simulink model "PMSM_motor"  (R2025b)
settings: Solver=VariableStepAuto  StartTime=0.0  StopTime=10  RelTol=1e-3
values from neighbouring files (symbols this model uses):
  p = 3    [task_run.m]    (also in task_run1.m; task_run2.m)
undefined symbols (not defined in the file or in its folder): Ld, Lq, omega_m_const, psi_f, Rs, theta_offset
libraries: fl_lib x10, nesl_utility x6, ee_lib x4
settings Model: Creator=Администратор  LastModifiedBy=Администратор

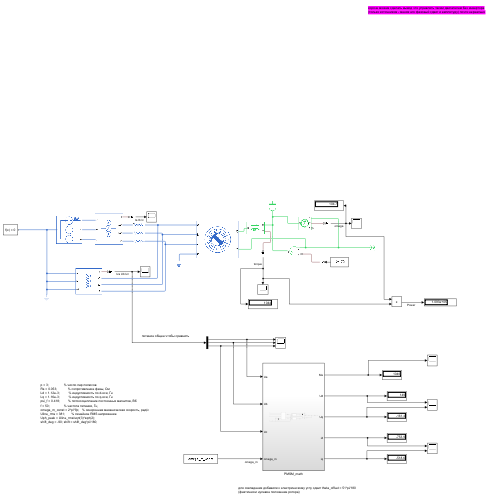
[thumbnail: Simulink's stored preview of the top-level diagram]
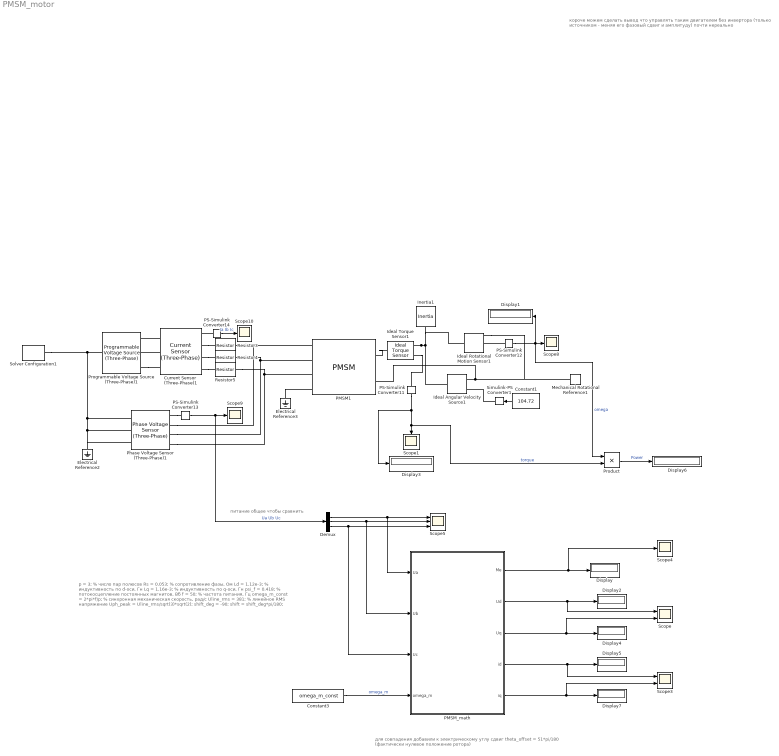
== system PMSM_motor ==
  note: для совпадения добавили к электрическому углу сдвиг theta_offset = 51*pi/180 (фактически нулевое положение ротора)
  note: питание общее чтобы сравнить
  note: p = 3;                 % число пар полюсов
      | Rs = 0.053;            % сопротивление фазы, Ом
      | Ld = 1.12e-3;          % индуктивность по d-оси, Гн
      | Lq = 1.16e-3;          % индуктивность по q-оси, Гн
      | psi_f = 0.418;         % потокосцепление постоянных магнитов, Вб
      | f = 50;                % частота питания, Гц
      | omega_m_const = 2*pi*f/p;   % синхронная механическая скорость, рад/с
      | Uline_rms = 381;       % линейное RMS напряжение
      | Uph_peak = Uline_rms/sqrt(3)*sqrt(2);
      | shift_deg = -90; shift = shift_deg*pi/180;
  note: короче можем сделать вывод что управлять таким двигателем без инвертора
      | (только источником - меняя его фазовый сдвиг и амплитуду) почти нереально
  Constant1 : Constant  Value=104.72
  Constant3 : Constant  Value=omega_m_const
  Current Sensor (Three-Phase)1 : ee_lib/Sensors & Transducers/Current Sensor (Three-Phase)
      settings: InternalSimscapePortConfiguration="{\"Bottom\":[],\"Left\":[{\"id\":\"a1\",\"label\":\"a1\",\"type\":\"foundation.electrical.electrical\"},{\"id\":\"b1\",\"label\":\"b1\",\"type\":\"foundation.electrical.electrical\"},{\"id\":\"c1\",\"label\":\"c1\",\"type\":\"foundation.electrical.electrical\"}],\"Right\":[{\"id\":\"I_output\",\"label\":\"I\",\"type\":\"output\"},{\"id\":\"a2\",\"label\":\"a2\",\"type\":\"foundation.electrical.electrical\"},{\"id\":\"b2\",\"label\":\"b2\",\"type\":\"foundation.electrical.electrical\"},{\"id\":\"c2\",\"label\":\"c2\",\"type\":\"foundation.electrical.electrical\"}],\"Top\":[]}"
  Demux : Demux  Outputs=3
  Display{,1..7} (8 alike) : Display
  Electrical Reference2 : fl_lib/Electrical/Electrical Elements/Electrical Reference
  Electrical Reference3 : fl_lib/Electrical/Electrical Elements/Electrical Reference
  Ideal Angular Velocity Source1 : fl_lib/Mechanical/Mechanical Sources/Ideal Angular Velocity Source
  Ideal Rotational Motion Sensor1 : fl_lib/Mechanical/Mechanical Sensors/Ideal Rotational Motion Sensor  reference=foundation.enum.MeasurementReference.difference  acceleration_port=false  velocity_port=true  position_port=true  wrap_angle=false  offset=0 rad
  Ideal Torque Sensor1 : fl_lib/Mechanical/Mechanical Sensors/Ideal Torque Sensor
  Inertia1 : fl_lib/Mechanical/Rotational Elements/Inertia  inertia=0.05 kg*m^2  num_ports=foundation.enum.numPorts2.one  w_specify=off  w_priority=High  w=0 rad/s  w_nominal_specify=off  w_nominal_value=1  w_nominal_unit=rad/s  t_specify=off  t_priority=None  t=0 N*m  t_nominal_specify=off  t_nominal_value=1  t_nominal_unit=N*m
  Mechanical Rotational Reference1 : fl_lib/Mechanical/Rotational Elements/Mechanical Rotational Reference
  PMSM1 : ee_lib/Electromechanical/Permanent Magnet/PMSM  port_option=ee.enum.threePhasePort.expanded  winding_type=ee.enum.electromech.statorconfiguration.wye  machine_param=ee.enum.pmsm.parameterization.constant  nPolePairs=3  pmflux_param=ee.enum.pmflux.fluxlinkage  pm_flux_linkage=0.418 Wb  torque_constant=0.18 N*m/A  back_emf_constant=0.18 V*s/rad  stator_param=ee.enum.statorparam.LdLqL0  Ld=1.12e-3 H  Lq=1.16e-3 H  idVec=[-200, 0, 200] A  iqVec=[-200, 0, 200] A  LdMatrix=0.0002 * ones(3, 3) H  LqMatrix=0.0002 * ones(3, 3) H  PmMatrix=0.1 * ones(3, 3) Wb  ktMatrix=0.18 * ones(3, 3) N*m/A  keMatrix=0.18 * ones(3, 3) V*s/rad  L0=0.005 H  Ls=0.0002 H  Lm=-0.00002 H  Ms=0.00002 H  Rs=0.053 Ohm  zero_sequence=ee.enum.park.zerosequence.include  axes_param=ee.enum.rotorangle.daxis  loss_param=ee.enum.ironloss.none  losses_oc=[0, 0, 0] W  losses_sc=[0, 0, 0] W  f_losses=60 Hz  Isc_losses=95 A  J=0.244 kg*m^2  lam=0.01 N*m*s/rad  i_d_specify=off  i_d_priority=None  i_d=0 A  i_d_nominal_specify=off  i_d_nominal_value=1  i_d_nominal_unit=A  i_q_specify=off  i_q_priority=None  i_q=0 A  i_q_nominal_specify=off  i_q_nominal_value=1  i_q_nominal_unit=A  torque_specify=off  torque_priority=None  torque=0 N*m  torque_nominal_specify=off  torque_nominal_value=1  torque_nominal_unit=N*m  angular_velocity_specify=off  angular_velocity_priority=High  angular_velocity=1000 rpm  angular_velocity_nominal_specify=off  angular_velocity_nominal_value=1  angular_velocity_nominal_unit=rpm  angular_position_specify=off  angular_position_priority=High  angular_position=-0 deg  angular_position_nominal_specify=off  angular_position_nominal_value=1  angular_position_nominal_unit=deg  alpha=3.93e-3 1/K  alpha_flux=-0.001 1/K  Tmeas=298.15 K  stator_thermal_mass=100 J/K  rotor_thermal_mass=200 J/K  Rm_percent_rotor=90  Rd_percent_rotor=30  temperatureA_specify=off  temperatureA_priority=High  temperatureA=25 degC  temperatureA_nominal_specify=off  temperatureA_nominal_value=1  temperatureA_nominal_unit=degC  temperatureB_specify=off  temperatureB_priority=High  temperatureB=25 degC  temperatureB_nominal_specify=off  temperatureB_nominal_value=1  temperatureB_nominal_unit=degC  temperatureC_specify=off  temperatureC_priority=High  temperatureC=25 degC  temperatureC_nominal_specify=off  temperatureC_nominal_value=1  temperatureC_nominal_unit=degC  temperatureR_specify=off  temperatureR_priority=High  temperatureR=25 degC  temperatureR_nominal_specify=off  temperatureR_nominal_value=1  temperatureR_nominal_unit=degC
      settings: InternalSimscapePortConfiguration="{\"Bottom\":[],\"Left\":[{\"id\":\"a\",\"label\":\"a\",\"type\":\"foundation.electrical.electrical\"},{\"id\":\"b\",\"label\":\"b\",\"type\":\"foundation.electrical.electrical\"},{\"id\":\"c\",\"label\":\"c\",\"type\":\"foundation.electrical.electrical\"},{\"id\":\"n\",\"label\":\"n\",\"type\":\"foundation.electrical.electrical\"}],\"Right\":[{\"id\":\"R\",\"label\":\"R\",\"type\":\"foundation.mechanical.rotational.rotational\"},{\"id\":\"C\",\"label\":\"C\",\"type\":\"foundation.mechanical.rotational.rotational\"}],\"Top\":[]}"
  PMSM_math : Subsystem
  PS-Simulink Converter{11..14} (4 alike) : nesl_utility/PS-Simulink Converter  PhysicalDomain=network_engine_domain  SubClassName=ps_output  LeftPortType=input  RightPortType=output  PseudoPeriodic=off  Frequencies=[]  VectorFormat=inherit  Unit=inherit  AffineConversion=off
  Phase Voltage Sensor (Three-Phase)1 : ee_lib/Sensors & Transducers/Phase Voltage Sensor (Three-Phase)
      settings: InternalSimscapePortConfiguration="{\"Bottom\":[],\"Left\":[{\"id\":\"a1\",\"label\":\"a1\",\"type\":\"foundation.electrical.electrical\"},{\"id\":\"b1\",\"label\":\"b1\",\"type\":\"foundation.electrical.electrical\"},{\"id\":\"c1\",\"label\":\"c1\",\"type\":\"foundation.electrical.electrical\"}],\"Right\":[{\"id\":\"V_output\",\"label\":\"V\",\"type\":\"output\"},{\"id\":\"a2\",\"label\":\"a2\",\"type\":\"foundation.electrical.electrical\"},{\"id\":\"b2\",\"label\":\"b2\",\"type\":\"foundation.electrical.electrical\"},{\"id\":\"c2\",\"label\":\"c2\",\"type\":\"foundation.electrical.electrical\"}],\"Top\":[]}"
  Product : Product
  Programmable Voltage Source (Three-Phase)1 : ee_lib/Sources/Programmable Voltage Source (Three-Phase)  magnitude_type=ee.enum.timechanging.constant  vline_rms=381 V  magn_ramp=1 V/s  magn_step=1 V  magn_modu_magn=1 V  magn_modu_freq=1 Hz  magn_t1=1 s  magn_t2=2 s  frequency_type=ee.enum.timechanging.constant  freq=50 Hz  freq_ramp=1 Hz/s  freq_step=1 Hz  freq_modu_magn=1 Hz  freq_modu_freq=1 Hz  freq_t1=1 s  freq_t2=2 s  phase_type=ee.enum.timechanging.constant  shift=shift_deg deg  phase_ramp=1 deg/s  phase_step=1 deg  phase_modu_magn=1 deg  phase_modu_freq=1 Hz  phase_t1=1 s  phase_t2=2 s  impedance_option=1  SShortCircuit=1e6 A*V  XR=15  R=0.01 Ohm  L=3.97e-4 H  G_parasitic=1e-6 1/Ohm  harmonic_option=0  harmonic_orders=[5, 7, 11, 13]  harmonic_ratios=[.1, .1, .1, .1]  harmonic_shifts=[0, 0, 0, 0] deg  harmonic_sequences=[1, 1, 1, 1]  harmonic_t1=-inf s  harmonic_t2=inf s  I_specify=off  I_priority=None  I=[0, 0, 0] A  I_nominal_specify=off  I_nominal_value=1  I_nominal_unit=A  V_specify=off  V_priority=None  V=[0, 0, 0] V  V_nominal_specify=off  V_nominal_value=1  V_nominal_unit=V
      settings: InternalSimscapePortConfiguration="{\"Bottom\":[],\"Left\":[{\"id\":\"n\",\"label\":\"n\",\"type\":\"foundation.electrical.electrical\"}],\"Right\":[{\"id\":\"a\",\"label\":\"a\",\"type\":\"foundation.electrical.electrical\"},{\"id\":\"b\",\"label\":\"b\",\"type\":\"foundation.electrical.electrical\"},{\"id\":\"c\",\"label\":\"c\",\"type\":\"foundation.electrical.electrical\"}],\"Top\":[]}"
  Resistor3 : fl_lib/Electrical/Electrical Elements/Resistor  R=0.0001 Ohm  i_specify=off  i_priority=None  i=0 A  i_nominal_specify=off  i_nominal_value=1  i_nominal_unit=A  v_specify=off  v_priority=None  v=0 V  v_nominal_specify=off  v_nominal_value=1  v_nominal_unit=V
  Resistor4 : fl_lib/Electrical/Electrical Elements/Resistor  R=0.0001 Ohm  i_specify=off  i_priority=None  i=0 A  i_nominal_specify=off  i_nominal_value=1  i_nominal_unit=A  v_specify=off  v_priority=None  v=0 V  v_nominal_specify=off  v_nominal_value=1  v_nominal_unit=V
  Resistor5 : fl_lib/Electrical/Electrical Elements/Resistor  R=0.0001 Ohm  i_specify=off  i_priority=None  i=0 A  i_nominal_specify=off  i_nominal_value=1  i_nominal_unit=A  v_specify=off  v_priority=None  v=0 V  v_nominal_specify=off  v_nominal_value=1  v_nominal_unit=V
  Scope : Scope  NumInputPorts=2
      settings: ActiveDisplayYMinimum=-350.30854261169594  ActiveDisplayYMaximum=38.547954055165228
  Scope{1,4,8..10} (5 alike) : Scope
      Scope1 settings: ActiveDisplayYMinimum=-2800.9306525300181  ActiveDisplayYMaximum=30125.951293394119  DataLoggingVariableName=ScopeData8
      Scope10 settings: ActiveDisplayYMinimum=-283.18935621511253  ActiveDisplayYMaximum=90.573418944669029  DataLoggingVariableName=ScopeData9
      Scope4 settings: ActiveDisplayYMinimum=1450.8447118873733  ActiveDisplayYMaximum=1641.0492571958657  DataLoggingVariableName=ScopeData3
      Scope8 settings: ActiveDisplayYMinimum=43.85278065599158  ActiveDisplayYMaximum=560.88321292559522  DataLoggingVariableName=ScopeData10
      Scope9 settings: ActiveDisplayYMinimum=-2097.2902957392048  ActiveDisplayYMaximum=438.53947123567758  DataLoggingVariableName=ScopeData11
  Scope3 : Scope  NumInputPorts=2
      settings: ActiveDisplayYMinimum=-688.36948573221423  ActiveDisplayYMaximum=823.2908720056123  DataLoggingVariableName=ScopeData2
  Scope5 : Scope  NumInputPorts=3
      settings: ActiveDisplayYMinimum=-50.251415686553713  ActiveDisplayYMaximum=426.06939710877936  DataLoggingVariableName=ScopeData4
  Simulink-PS Converter1 : nesl_utility/Simulink-PS Converter  PhysicalDomain=network_engine_domain  SubClassName=ps_input  LeftPortType=input  RightPortType=output  PseudoPeriodic=off  Frequencies=[]  NoiseDistribution=none  NoiseParameters=[]  Unit=rad/s  AffineConversion=off  FilteringAndDerivatives=provide  SimscapeFilterOrder=1  InputFilterTimeConstant=0.001  UdotUserProvided=0
  Solver Configuration1 : nesl_utility/Solver Configuration  PhysicalDomain=network_engine_domain  SubClassName=solver  LeftPortType=input  RightPortType=generic  Tones=[]  Harmonics=[]  SimulateNoise=off  Profile=off  UseLocalSampling=off  EnableSwitchedLinearOptims=on  FrequencyDomain=off  UseCCode=off  RelTol=0.001  AbsTol=0.001  MinStep=1e-09  ToWorkspace=off  RevertToSquareIcSolve=off  NumHomotopyIterations=100  PhasorMode=off  PhasorModeNumHarmonics=1  ConsistencySolver=NEWTON_XTOL_AFTER_FTOL  IndexReductionMethod=DerivativeReplacement  DoDC=off  ResidualTolerance=1e-09  ConsistencyTolSource=GLOBAL  ConsistencyAbsTol=0.001  ConsistencyRelTol=0.001  ConsistencyTolFactor=0.001  UseLocalSolver=off  LocalSolverChoice=NE_BACKWARD_EULER_ADVANCER  ResolveIndetEquations=on  FunctionEvalNumThread=1  LocalSolverSampleTime=0.001  DoFixedCost=off  MaxNonlinIter=3  MaxModeIter=2  ComputeImpulses=off  ImpulseIterations=2  LinearAlgebra=auto  LinearAlgebraNumThread=0  EquationFormulation=NE_TIME_EF  DelaysMemoryBudget=1024  AutomaticFiltering=on  FilteringTimeConstant=0.001  PartitionStorageMethod=AS_NEEDED  PartitionMemoryBudget=1024  PartitionMethod=ROBUST  MultibodyUseLocalSolver=off  MultibodyLocalSolverChoice=ODE1  MultibodyLocalSolverSampleTime=0.001
  wires:
  PS-Simulink Converter11/1 -> Product/2, Scope1/1, Display3/1  "torque"
  Product/1 -> Display6/1  "Power"
  PS-Simulink Converter14/1 -> Scope10/1  "Ia Ib Ic"
  PS-Simulink Converter12/1 -> Product/1, Display1/1, Scope8/1  "omega"
  Constant1/1 -> Simulink-PS Converter1/1
  PS-Simulink Converter13/1 -> Demux/1, Scope9/1  "Ua Ub Uc"
  Constant3/1 -> PMSM_math/4(omega_m)  "omega_m"
  PMSM_math/2(Ud) -> Display2/1, Scope/1
  PMSM_math/3(Uq) -> Display4/1, Scope/2
  PMSM_math/4(id) -> Display5/1, Scope3/1
  PMSM_math/5(iq) -> Display7/1, Scope3/2
  PMSM_math/1(Me) -> Display/1, Scope4/1
  Demux/1 -> Scope5/1, PMSM_math/1(Ua)
  Demux/2 -> PMSM_math/2(Ub), Scope5/2
  Demux/3 -> PMSM_math/3(Uc), Scope5/3
  connections:
  Phase Voltage Sensor (Three-Phase)1/LConn2 -- Electrical Reference2/LConn1 -- Phase Voltage Sensor (Three-Phase)1/LConn3 -- Solver Configuration1/RConn1 -- Programmable Voltage Source (Three-Phase)1/LConn1 -- Phase Voltage Sensor (Three-Phase)1/LConn1
  Ideal Angular Velocity Source1/RConn2 -- Ideal Rotational Motion Sensor1/RConn1 -- Mechanical Rotational Reference1/LConn1 -- PMSM1/RConn2
  Current Sensor (Three-Phase)1/RConn4 -- Resistor5/LConn1
  Ideal Torque Sensor1/RConn1 -- Ideal Rotational Motion Sensor1/LConn1 -- Inertia1/LConn1 -- Ideal Angular Velocity Source1/LConn1
  Current Sensor (Three-Phase)1/RConn2 -- Resistor3/LConn1
  Phase Voltage Sensor (Three-Phase)1/RConn3 -- Resistor4/RConn1 -- PMSM1/LConn2
  Current Sensor (Three-Phase)1/LConn2 -- Programmable Voltage Source (Three-Phase)1/RConn2
  PS-Simulink Converter14/LConn1 -- Current Sensor (Three-Phase)1/RConn1
  Phase Voltage Sensor (Three-Phase)1/RConn1 -- PS-Simulink Converter13/LConn1
  Ideal Torque Sensor1/RConn2 -- PS-Simulink Converter11/LConn1
  Ideal Torque Sensor1/LConn1 -- PMSM1/RConn1
  Programmable Voltage Source (Three-Phase)1/RConn3 -- Current Sensor (Three-Phase)1/LConn3
  Current Sensor (Three-Phase)1/LConn1 -- Programmable Voltage Source (Three-Phase)1/RConn1
  PS-Simulink Converter12/LConn1 -- Ideal Rotational Motion Sensor1/RConn2
  Simulink-PS Converter1/RConn1 -- Ideal Angular Velocity Source1/RConn1
  Electrical Reference3/LConn1 -- PMSM1/LConn4
  Resistor3/RConn1 -- Phase Voltage Sensor (Three-Phase)1/RConn2 -- PMSM1/LConn1
  Current Sensor (Three-Phase)1/RConn3 -- Resistor4/LConn1
  Resistor5/RConn1 -- Phase Voltage Sensor (Three-Phase)1/RConn4 -- PMSM1/LConn3

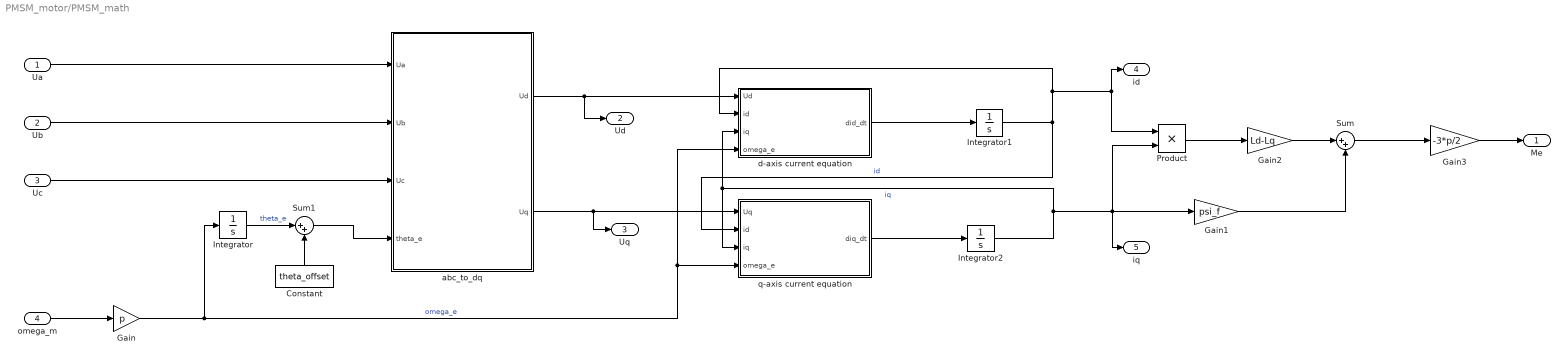
== system PMSM_motor/PMSM_math ==
  Ua : Inport
  Ub : Inport  Port=2
  Uc : Inport  Port=3
  omega_m : Inport  Port=4
  Constant : Constant  Value=theta_offset
  Gain : Gain  Gain=p
  Gain1 : Gain  Gain=psi_f
  Gain2 : Gain  Gain=Ld-Lq
  Gain3 : Gain  Gain=-3*p/2
  Integrator : Integrator
  Integrator1 : Integrator
  Integrator2 : Integrator
  Product : Product
  Sum : Sum  Inputs=|++
  Sum1 : Sum  Inputs=|++
  abc_to_dq : Subsystem
  d-axis current equation : Subsystem
  q-axis current equation : Subsystem
  Me : Outport
  Ud : Outport  Port=2
  Uq : Outport  Port=3
  id : Outport  Port=4
  iq : Outport  Port=5
  wires:
  omega_m/1 -> Gain/1
  Gain/1 -> d-axis current equation/4(omega_e), q-axis current equation/4(omega_e), Integrator/1  "omega_e"
  Integrator/1 -> Sum1/1  "theta_e"
  Ua/1 -> abc_to_dq/1(Ua)
  Ub/1 -> abc_to_dq/2(Ub)
  Uc/1 -> abc_to_dq/3(Uc)
  abc_to_dq/1(Ud) -> d-axis current equation/1(Ud), Ud/1
  abc_to_dq/2(Uq) -> q-axis current equation/1(Uq), Uq/1
  d-axis current equation/1(did_dt) -> Integrator1/1
  q-axis current equation/1(diq_dt) -> Integrator2/1
  Integrator1/1 -> Product/1, id/1, d-axis current equation/2(id), q-axis current equation/2(id)  "id"
  Integrator2/1 -> d-axis current equation/3(iq), q-axis current equation/3(iq), Product/2, iq/1, Gain1/1  "iq"
  Product/1 -> Gain2/1
  Gain2/1 -> Sum/1
  Gain3/1 -> Me/1
  Gain1/1 -> Sum/2
  Sum/1 -> Gain3/1
  Sum1/1 -> abc_to_dq/4(theta_e)
  Constant/1 -> Sum1/2

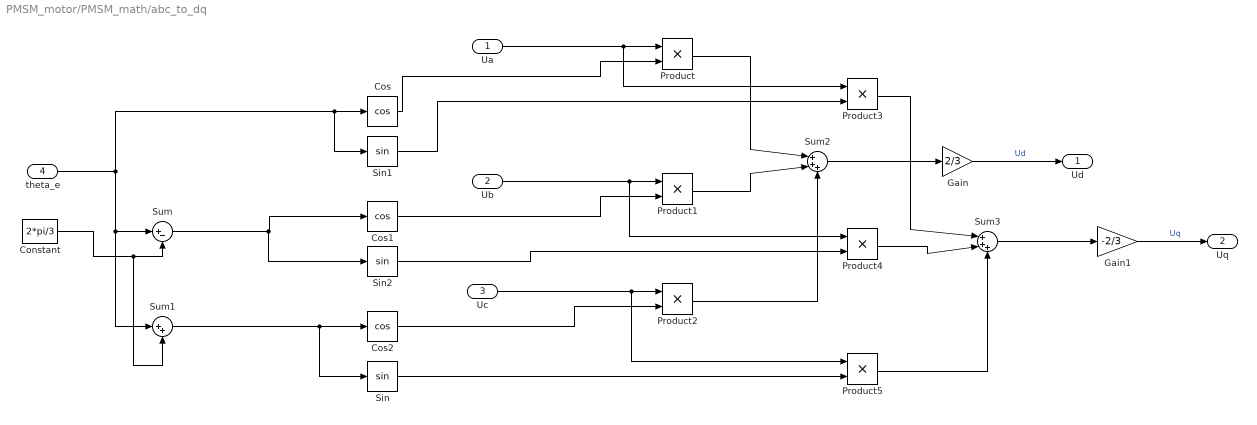
== system PMSM_motor/PMSM_math/abc_to_dq ==
  Ua : Inport
  Ub : Inport  Port=2
  Uc : Inport  Port=3
  theta_e : Inport  Port=4
  Constant : Constant  Value=2*pi/3
  Cos : Trigonometry  Operator=cos
  Cos1 : Trigonometry  Operator=cos
  Cos2 : Trigonometry  Operator=cos
  Gain : Gain  Gain=2/3
  Gain1 : Gain  Gain=-2/3
  Product{,1..5} (6 alike) : Product
  Sin : Trigonometry
  Sin1 : Trigonometry
  Sin2 : Trigonometry
  Sum : Sum  Inputs=|+-
  Sum1 : Sum  Inputs=|++
  Sum2 : Sum  Inputs=|+++
  Sum3 : Sum  Inputs=|+++
  Ud : Outport
  Uq : Outport  Port=2
  wires:
  theta_e/1 -> Sum1/1, Sum/1, Sin1/1, Cos/1
  Constant/1 -> Sum1/2, Sum/2
  Cos/1 -> Product/2
  Ua/1 -> Product3/1, Product/1
  Sum/1 -> Sin2/1, Cos1/1
  Ub/1 -> Product4/1, Product1/1
  Sum1/1 -> Sin/1, Cos2/1
  Uc/1 -> Product5/1, Product2/1
  Cos1/1 -> Product1/2
  Cos2/1 -> Product2/2
  Product/1 -> Sum2/1
  Product1/1 -> Sum2/2
  Product2/1 -> Sum2/3
  Sum2/1 -> Gain/1
  Gain/1 -> Ud/1  "Ud"
  Sin1/1 -> Product3/2
  Sin2/1 -> Product4/2
  Sin/1 -> Product5/2
  Product3/1 -> Sum3/1
  Product4/1 -> Sum3/2
  Product5/1 -> Sum3/3
  Sum3/1 -> Gain1/1
  Gain1/1 -> Uq/1  "Uq"

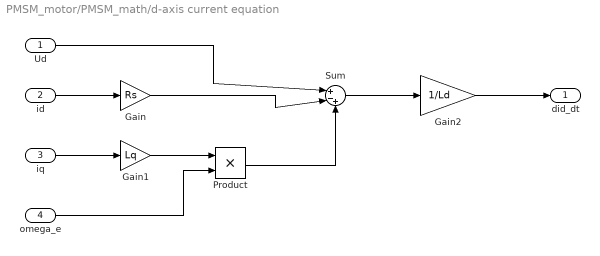
== system PMSM_motor/PMSM_math/d-axis current equation ==
  Ud : Inport
  id : Inport  Port=2
  iq : Inport  Port=3
  omega_e : Inport  Port=4
  Gain : Gain  Gain=Rs
  Gain1 : Gain  Gain=Lq
  Gain2 : Gain  Gain=1/Ld
  Product : Product
  Sum : Sum  Inputs=|+-+
  did_dt : Outport
  wires:
  id/1 -> Gain/1
  iq/1 -> Gain1/1
  Gain1/1 -> Product/1
  omega_e/1 -> Product/2
  Ud/1 -> Sum/1
  Gain/1 -> Sum/2
  Product/1 -> Sum/3
  Sum/1 -> Gain2/1
  Gain2/1 -> did_dt/1

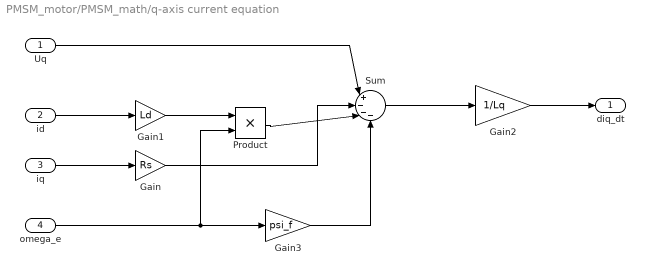
== system PMSM_motor/PMSM_math/q-axis current equation ==
  Uq : Inport
  id : Inport  Port=2
  iq : Inport  Port=3
  omega_e : Inport  Port=4
  Gain : Gain  Gain=Rs
  Gain1 : Gain  Gain=Ld
  Gain2 : Gain  Gain=1/Lq
  Gain3 : Gain  Gain=psi_f
  Product : Product
  Sum : Sum  Inputs=|+---
  diq_dt : Outport
  wires:
  omega_e/1 -> Gain3/1, Product/2
  Gain/1 -> Sum/2
  Uq/1 -> Sum/1
  Sum/1 -> Gain2/1
  Gain2/1 -> diq_dt/1
  id/1 -> Gain1/1
  Product/1 -> Sum/3
  iq/1 -> Gain/1
  Gain1/1 -> Product/1
  Gain3/1 -> Sum/4
